simulink model "vss_model"  (R2016b)
settings: Solver=FixedStepDiscrete  StartTime=0.0  StopTime=10.0  FixedStep=0.01  RelTol=1e-3
libraries: simulink x2
settings Model: Creator=Borja Martos  LastModifiedBy=Borja Martos

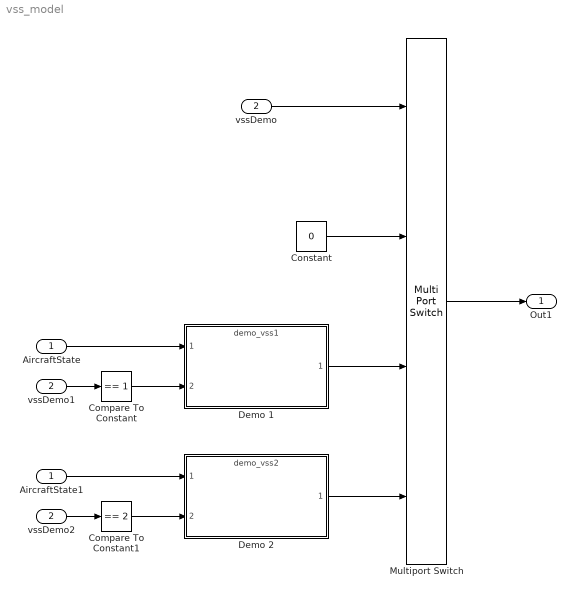
== system vss_model ==
  AircraftState : Inport  OutDataTypeStr=Bus: INPUTS
  vssDemo : Inport  Port=2
  AircraftState1 : InportShadow  OutDataTypeStr=Bus: INPUTS
  Compare To Constant : simulink/Logic and Bit Operations/Compare To Constant  relop===  const=1  OutDataTypeStr=boolean
  Compare To Constant1 : simulink/Logic and Bit Operations/Compare To Constant  relop===  const=2  OutDataTypeStr=boolean
  Constant : Constant  Value=0
  Demo 1 : ModelReference  ModelNameDialog=demo_vss1.slx  SimulationMode=Normal  ModelReferenceVersion=1.8
  Demo 2 : ModelReference  ModelNameDialog=demo_vss2.slx  SimulationMode=Normal  ModelReferenceVersion=1.9
  Multiport Switch : MultiPortSwitch  DataPortOrder=Zero-based contiguous  DiagnosticForDefault=None
  vssDemo1 : InportShadow  Port=2
  vssDemo2 : InportShadow  Port=2
  Out1 : Outport
  wires:
  AircraftState/1 -> Demo 1/1
  vssDemo1/1 -> Compare To Constant/1
  Compare To Constant/1 -> Demo 1/2
  AircraftState1/1 -> Demo 2/1
  vssDemo2/1 -> Compare To Constant1/1
  Compare To Constant1/1 -> Demo 2/2
  Demo 2/1 -> Multiport Switch/4
  vssDemo/1 -> Multiport Switch/1
  Multiport Switch/1 -> Out1/1
  Demo 1/1 -> Multiport Switch/3
  Constant/1 -> Multiport Switch/2
